simulink model "Model"  (R2023b)
settings: Solver=FixedStepAuto  StartTime=0.0  StopTime=10  FixedStep=0.002  RelTol=1e-3
model workspace (MAT data in the model file):
  a = 0
undefined symbols (not defined in the file or in its folder): X, Y, Z
libraries: sm_lib x84, nesl_utility x29, slpidlib x9, simulink x6
(part 6 of 7)

== matlab function Model/左腿VMC ==
  data: phi_1 input; phi_4 input; F input; T1 output; T2 output; Tp input
function [T1,T2]= fcn(phi_1,phi_4,F,Tp)

l_1=0.15;
l_2=0.27;
l_3=0.27;
l_4=0.15;
l_5=0.15;

J11=(2*(l_1*cos(phi_1) + (2*l_2*cos(2*atan(((4*l_2^2*(l_1*sin(phi_1) - l_4*sin(phi_4))^2 - ((l_1*sin(phi_1) - l_4*sin(phi_4))^2 + (l_5 - l_1*cos(phi_1) + l_4*cos(phi_4))^2 + l_2^2 - l_3^2)^2 + 4*l_2^2*(l_5 - l_1*cos(phi_1) + l_4*cos(phi_4))^2)^(1/2) - 2*l_2*(l_1*sin(phi_1) - l_4*sin(phi_4)))/((l_1*sin(phi_1) - l_4*sin(phi_4))^2 + (l_5 - l_1*cos(phi_1) + l_4*cos(phi_4))^2 + l_2^2 - l_3^2 + 2*l_2*(l_5 - l_1*cos(phi_1) + l_4*cos(phi_4)))))*(((8*l_1*l_2^2*cos(phi_1)*(l_1*sin(phi_1) - l_4*sin(phi_4)) - 2*(2*l_1*cos(phi_1)*(l_1*sin(phi_1) - l_4*sin(phi_4)) + 2*l_1*sin(phi_1)*(l_5 - l_1*cos(phi_1) + l_4*cos(phi_4)))*((l_1*sin(phi_1) - l_4*sin(phi_4))^2 + (l_5 - l_1*cos(phi_1) + l_4*cos(phi_4))^2 + l_2^2 - l_3^2) + 8*l_1*l_2^2*sin(phi_1)*(l_5 - l_1*cos(phi_1) + l_4*cos(phi_4)))/(2*(4*l_2^2*(l_1*sin(phi_1) - l_4*sin(phi_4))^2 - ((l_1*sin(phi_1) - l_4*sin(phi_4))^2 + (l_5 - l_1*cos(phi_1) + l_4*cos(phi_4))^2 + l_2^2 - l_3^2)^2 + 4*l_2^2*(l_5 - l_1*cos(phi_1) + l_4*cos(phi_4))^2)^(1/2)) - 2*l_1*l_2*cos(phi_1))/((l_1*sin(phi_1) - l_4*sin(phi_4))^2 + (l_5 - l_1*cos(phi_1) + l_4*cos(phi_4))^2 + l_2^2 - l_3^2 + 2*l_2*(l_5 - l_1*cos(phi_1) + l_4*cos(phi_4))) - (((4*l_2^2*(l_1*sin(phi_1) - l_4*sin(phi_4))^2 - ((l_1*sin(phi_1) - l_4*sin(phi_4))^2 + (l_5 - l_1*cos(phi_1) + l_4*cos(phi_4))^2 + l_2^2 - l_3^2)^2 + 4*l_2^2*(l_5 - l_1*cos(phi_1) + l_4*cos(phi_4))^2)^(1/2) - 2*l_2*(l_1*sin(phi_1) - l_4*sin(phi_4)))*(2*l_1*l_2*sin(phi_1) + 2*l_1*cos(phi_1)*(l_1*sin(phi_1) - l_4*sin(phi_4)) + 2*l_1*sin(phi_1)*(l_5 - l_1*cos(phi_1) + l_4*cos(phi_4))))/((l_1*sin(phi_1) - l_4*sin(phi_4))^2 + (l_5 - l_1*cos(phi_1) + l_4*cos(phi_4))^2 + l_2^2 - l_3^2 + 2*l_2*(l_5 - l_1*cos(phi_1) + l_4*cos(phi_4)))^2))/(((4*l_2^2*(l_1*sin(phi_1) - l_4*sin(phi_4))^2 - ((l_1*sin(phi_1) - l_4*sin(phi_4))^2 + (l_5 - l_1*cos(phi_1) + l_4*cos(phi_4))^2 + l_2^2 - l_3^2)^2 + 4*l_2^2*(l_5 - l_1*cos(phi_1) + l_4*cos(phi_4))^2)^(1/2) - 2*l_2*(l_1*sin(phi_1) - l_4*sin(phi_4)))^2/((l_1*sin(phi_1) - l_4*sin(phi_4))^2 + (l_5 - l_1*cos(phi_1) + l_4*cos(phi_4))^2 + l_2^2 - l_3^2 + 2*l_2*(l_5 - l_1*cos(phi_1) + l_4*cos(phi_4)))^2 + 1))*(l_2*sin(2*atan(((4*l_2^2*(l_1*sin(phi_1) - l_4*sin(phi_4))^2 - ((l_1*sin(phi_1) - l_4*sin(phi_4))^2 + (l_5 - l_1*cos(phi_1) + l_4*cos(phi_4))^2 + l_2^2 - l_3^2)^2 + 4*l_2^2*(l_5 - l_1*cos(phi_1) + l_4*cos(phi_4))^2)^(1/2) - 2*l_2*(l_1*sin(phi_1) - l_4*sin(phi_4)))/((l_1*sin(phi_1) - l_4*sin(phi_4))^2 + (l_5 - l_1*cos(phi_1) + l_4*cos(phi_4))^2 + l_2^2 - l_3^2 + 2*l_2*(l_5 - l_1*cos(phi_1) + l_4*cos(phi_4))))) + l_1*sin(phi_1)) - 2*(l_1*sin(phi_1) + (2*l_2*sin(2*atan(((4*l_2^2*(l_1*sin(phi_1) - l_4*sin(phi_4))^2 - ((l_1*sin(phi_1) - l_4*sin(phi_4))^2 + (l_5 - l_1*cos(phi_1) + l_4*cos(phi_4))^2 + l_2^2 - l_3^2)^2 + 4*l_2^2*(l_5 - l_1*cos(phi_1) + l_4*cos(phi_4))^2)^(1/2) - 2*l_2*(l_1*sin(phi_1) - l_4*sin(phi_4)))/((l_1*sin(phi_1) - l_4*sin(phi_4))^2 + (l_5 - l_1*cos(phi_1) + l_4*cos(phi_4))^2 + l_2^2 - l_3^2 + 2*l_2*(l_5 - l_1*cos(phi_1) + l_4*cos(phi_4)))))*(((8*l_1*l_2^2*cos(phi_1)*(l_1*sin(phi_1) - l_4*sin(phi_4)) - 2*(2*l_1*cos(phi_1)*(l_1*sin(phi_1) - l_4*sin(phi_4)) + 2*l_1*sin(phi_1)*(l_5 - l_1*cos(phi_1) + l_4*cos(phi_4)))*((l_1*sin(phi_1) - l_4*sin(phi_4))^2 + (l_5 - l_1*cos(phi_1) + l_4*cos(phi_4))^2 + l_2^2 - l_3^2) + 8*l_1*l_2^2*sin(phi_1)*(l_5 - l_1*cos(phi_1) + l_4*cos(phi_4)))/(2*(4*l_2^2*(l_1*sin(phi_1) - l_4*sin(phi_4))^2 - ((l_1*sin(phi_1) - l_4*sin(phi_4))^2 + (l_5 - l_1*cos(phi_1) + l_4*cos(phi_4))^2 + l_2^2 - l_3^2)^2 + 4*l_2^2*(l_5 - l_1*cos(phi_1) + l_4*cos(phi_4))^2)^(1/2)) - 2*l_1*l_2*cos(phi_1))/((l_1*sin(phi_1) - l_4*sin(phi_4))^2 + (l_5 - l_1*cos(phi_1) + l_4*cos(phi_4))^2 + l_2^2 - l_3^2 + 2*l_2*(l_5 - l_1*cos(phi_1) + l_4*cos(phi_4))) - (((4*l_2^2*(l_1*sin(phi_1) - l_4*sin(phi_4))^2 - ((l_1*sin(phi_1) - l_4*sin(phi_4))^2 + (l_5 - l_1*cos(phi_1) + l_4*cos(phi_4))^2 + l_2^2 - l_3^2)^2 + 4*l_2^2*(l_5 - l_1*cos(phi_1) + l_4*cos(phi_4))^2)^(1/2) - 2*l_2*(l_1*sin(phi_1) - l_4*sin(phi_4)))*(2*l_1*l_2*sin(phi_1) + 2*l_1*cos(phi_1)*(l_1*sin(phi_1) - l_4*sin(phi_4)) + 2*l_1*sin(phi_1)*(l_5 - l_1*cos(phi_1) + l_4*cos(phi_4))))/((l_1*sin(phi_1) - l_4*sin(phi_4))^2 + (l_5 - l_1*cos(phi_1) + l_4*cos(phi_4))^2 + l_2^2 - l_3^2 + 2*l_2*(l_5 - l_1*cos(phi_1) + l_4*cos(phi_4)))^2))/(((4*l_2^2*(l_1*sin(phi_1) - l_4*sin(phi_4))^2 - ((l_1*sin(phi_1) - l_4*sin(phi_4))^2 + (l_5 - l_1*cos(phi_1) + l_4*cos(phi_4))^2 + l_2^2 - l_3^2)^2 + 4*l_2^2*(l_5 - l_1*cos(phi_1) + l_4*cos(phi_4))^2)^(1/2) - 2*l_2*(l_1*sin(phi_1) - l_4*sin(phi_4)))^2/((l_1*sin(phi_1) - l_4*sin(phi_4))^2 + (l_5 - l_1*cos(phi_1) + l_4*cos(phi_4))^2 + l_2^2 - l_3^2 + 2*l_2*(l_5 - l_1*cos(phi_1) + l_4*cos(phi_4)))^2 + 1))*(l_2*cos(2*atan(((4*l_2^2*(l_1*sin(phi_1) - l_4*sin(phi_4))^2 - ((l_1*sin(phi_1) - l_4*sin(phi_4))^2 + (l_5 - l_1*cos(phi_1) + l_4*cos(phi_4))^2 + l_2^2 - l_3^2)^2 + 4*l_2^2*(l_5 - l_1*cos(phi_1) + l_4*cos(phi_4))^2)^(1/2) - 2*l_2*(l_1*sin(phi_1) - l_4*sin(phi_4)))/((l_1*sin(phi_1) - l_4*sin(phi_4))^2 + (l_5 - l_1*cos(phi_1) + l_4*cos(phi_4))^2 + l_2^2 - l_3^2 + 2*l_2*(l_5 - l_1*cos(phi_1) + l_4*cos(phi_4))))) - l_5/2 + l_1*cos(phi_1)))/(2*((l_2*sin(2*atan(((4*l_2^2*(l_1*sin(phi_1) - l_4*sin(phi_4))^2 - ((l_1*sin(phi_1) - l_4*sin(phi_4))^2 + (l_5 - l_1*cos(phi_1) + l_4*cos(phi_4))^2 + l_2^2 - l_3^2)^2 + 4*l_2^2*(l_5 - l_1*cos(phi_1) + l_4*cos(phi_4))^2)^(1/2) - 2*l_2*(l_1*sin(phi_1) - l_4*sin(phi_4)))/((l_1*sin(phi_1) - l_4*sin(phi_4))^2 + (l_5 - l_1*cos(phi_1) + l_4*cos(phi_4))^2 + l_2^2 - l_3^2 + 2*l_2*(l_5 - l_1*cos(phi_1) + l_4*cos(phi_4))))) + l_1*sin(phi_1))^2 + (l_2*cos(2*atan(((4*l_2^2*(l_1*sin(phi_1) - l_4*sin(phi_4))^2 - ((l_1*sin(phi_1) - l_4*sin(phi_4))^2 + (l_5 - l_1*cos(phi_1) + l_4*cos(phi_4))^2 + l_2^2 - l_3^2)^2 + 4*l_2^2*(l_5 - l_1*cos(phi_1) + l_4*cos(phi_4))^2)^(1/2) - 2*l_2*(l_1*sin(phi_1) - l_4*sin(phi_4)))/((l_1*sin(phi_1) - l_4*sin(phi_4))^2 + (l_5 - l_1*cos(phi_1) + l_4*cos(phi_4))^2 + l_2^2 - l_3^2 + 2*l_2*(l_5 - l_1*cos(phi_1) + l_4*cos(phi_4))))) - l_5/2 + l_1*cos(phi_1))^2)^(1/2));
J12=((4*l_2*sin(2*atan(((4*l_2^2*(l_1*sin(phi_1) - l_4*sin(phi_4))^2 - ((l_1*sin(phi_1) - l_4*sin(phi_4))^2 + (l_5 - l_1*cos(phi_1) + l_4*cos(phi_4))^2 + l_2^2 - l_3^2)^2 + 4*l_2^2*(l_5 - l_1*cos(phi_1) + l_4*cos(phi_4))^2)^(1/2) - 2*l_2*(l_1*sin(phi_1) - l_4*sin(phi_4)))/((l_1*sin(phi_1) - l_4*sin(phi_4))^2 + (l_5 - l_1*cos(phi_1) + l_4*cos(phi_4))^2 + l_2^2 - l_3^2 + 2*l_2*(l_5 - l_1*cos(phi_1) + l_4*cos(phi_4)))))*(((8*l_2^2*l_4*cos(phi_4)*(l_1*sin(phi_1) - l_4*sin(phi_4)) - 2*(2*l_4*cos(phi_4)*(l_1*sin(phi_1) - l_4*sin(phi_4)) + 2*l_4*sin(phi_4)*(l_5 - l_1*cos(phi_1) + l_4*cos(phi_4)))*((l_1*sin(phi_1) - l_4*sin(phi_4))^2 + (l_5 - l_1*cos(phi_1) + l_4*cos(phi_4))^2 + l_2^2 - l_3^2) + 8*l_2^2*l_4*sin(phi_4)*(l_5 - l_1*cos(phi_1) + l_4*cos(phi_4)))/(2*(4*l_2^2*(l_1*sin(phi_1) - l_4*sin(phi_4))^2 - ((l_1*sin(phi_1) - l_4*sin(phi_4))^2 + (l_5 - l_1*cos(phi_1) + l_4*cos(phi_4))^2 + l_2^2 - l_3^2)^2 + 4*l_2^2*(l_5 - l_1*cos(phi_1) + l_4*cos(phi_4))^2)^(1/2)) - 2*l_2*l_4*cos(phi_4))/((l_1*sin(phi_1) - l_4*sin(phi_4))^2 + (l_5 - l_1*cos(phi_1) + l_4*cos(phi_4))^2 + l_2^2 - l_3^2 + 2*l_2*(l_5 - l_1*cos(phi_1) + l_4*cos(phi_4))) - (((4*l_2^2*(l_1*sin(phi_1) - l_4*sin(phi_4))^2 - ((l_1*sin(phi_1) - l_4*sin(phi_4))^2 + (l_5 - l_1*cos(phi_1) + l_4*cos(phi_4))^2 + l_2^2 - l_3^2)^2 + 4*l_2^2*(l_5 - l_1*cos(phi_1) + l_4*cos(phi_4))^2)^(1/2) - 2*l_2*(l_1*sin(phi_1) - l_4*sin(phi_4)))*(2*l_2*l_4*sin(phi_4) + 2*l_4*cos(phi_4)*(l_1*sin(phi_1) - l_4*sin(phi_4)) + 2*l_4*sin(phi_4)*(l_5 - l_1*cos(phi_1) + l_4*cos(phi_4))))/((l_1*sin(phi_1) - l_4*sin(phi_4))^2 + (l_5 - l_1*cos(phi_1) + l_4*cos(phi_4))^2 + l_2^2 - l_3^2 + 2*l_2*(l_5 - l_1*cos(phi_1) + l_4*cos(phi_4)))^2)*(l_2*cos(2*atan(((4*l_2^2*(l_1*sin(phi_1) - l_4*sin(phi_4))^2 - ((l_1*sin(phi_1) - l_4*sin(phi_4))^2 + (l_5 - l_1*cos(phi_1) + l_4*cos(phi_4))^2 + l_2^2 - l_3^2)^2 + 4*l_2^2*(l_5 - l_1*cos(phi_1) + l_4*cos(phi_4))^2)^(1/2) - 2*l_2*(l_1*sin(phi_1) - l_4*sin(phi_4)))/((l_1*sin(phi_1) - l_4*sin(phi_4))^2 + (l_5 - l_1*cos(phi_1) + l_4*cos(phi_4))^2 + l_2^2 - l_3^2 + 2*l_2*(l_5 - l_1*cos(phi_1) + l_4*cos(phi_4))))) - l_5/2 + l_1*cos(phi_1)))/(((4*l_2^2*(l_1*sin(phi_1) - l_4*sin(phi_4))^2 - ((l_1*sin(phi_1) - l_4*sin(phi_4))^2 + (l_5 - l_1*cos(phi_1) + l_4*cos(phi_4))^2 + l_2^2 - l_3^2)^2 + 4*l_2^2*(l_5 - l_1*cos(phi_1) + l_4*cos(phi_4))^2)^(1/2) - 2*l_2*(l_1*sin(phi_1) - l_4*sin(phi_4)))^2/((l_1*sin(phi_1) - l_4*sin(phi_4))^2 + (l_5 - l_1*cos(phi_1) + l_4*cos(phi_4))^2 + l_2^2 - l_3^2 + 2*l_2*(l_5 - l_1*cos(phi_1) + l_4*cos(phi_4)))^2 + 1) - (4*l_2*cos(2*atan(((4*l_2^2*(l_1*sin(phi_1) - l_4*sin(phi_4))^2 - ((l_1*sin(phi_1) - l_4*sin(phi_4))^2 + (l_5 - l_1*cos(phi_1) + l_4*cos(phi_4))^2 + l_2^2 - l_3^2)^2 + 4*l_2^2*(l_5 - l_1*cos(phi_1) + l_4*cos(phi_4))^2)^(1/2) - 2*l_2*(l_1*sin(phi_1) - l_4*sin(phi_4)))/((l_1*sin(phi_1) - l_4*sin(phi_4))^2 + (l_5 - l_1*cos(phi_1) + l_4*cos(phi_4))^2 + l_2^2 - l_3^2 + 2*l_2*(l_5 - l_1*cos(phi_1) + l_4*cos(phi_4)))))*(l_2*sin(2*atan(((4*l_2^2*(l_1*sin(phi_1) - l_4*sin(phi_4))^2 - ((l_1*sin(phi_1) - l_4*sin(phi_4))^2 + (l_5 - l_1*cos(phi_1) + l_4*cos(phi_4))^2 + l_2^2 - l_3^2)^2 + 4*l_2^2*(l_5 - l_1*cos(phi_1) + l_4*cos(phi_4))^2)^(1/2) - 2*l_2*(l_1*sin(phi_1) - l_4*sin(phi_4)))/((l_1*sin(phi_1) - l_4*sin(phi_4))^2 + (l_5 - l_1*cos(phi_1) + l_4*cos(phi_4))^2 + l_2^2 - l_3^2 + 2*l_2*(l_5 - l_1*cos(phi_1) + l_4*cos(phi_4))))) + l_1*sin(phi_1))*(((8*l_2^2*l_4*cos(phi_4)*(l_1*sin(phi_1) - l_4*sin(phi_4)) - 2*(2*l_4*cos(phi_4)*(l_1*sin(phi_1) - l_4*sin(phi_4)) + 2*l_4*sin(phi_4)*(l_5 - l_1*cos(phi_1) + l_4*cos(phi_4)))*((l_1*sin(phi_1) - l_4*sin(phi_4))^2 + (l_5 - l_1*cos(phi_1) + l_4*cos(phi_4))^2 + l_2^2 - l_3^2) + 8*l_2^2*l_4*sin(phi_4)*(l_5 - l_1*cos(phi_1) + l_4*cos(phi_4)))/(2*(4*l_2^2*(l_1*sin(phi_1) - l_4*sin(phi_4))^2 - ((l_1*sin(phi_1) - l_4*sin(phi_4))^2 + (l_5 - l_1*cos(phi_1) + l_4*cos(phi_4))^2 + l_2^2 - l_3^2)^2 + 4*l_2^2*(l_5 - l_1*cos(phi_1) + l_4*cos(phi_4))^2)^(1/2)) - 2*l_2*l_4*cos(phi_4))/((l_1*sin(phi_1) - l_4*sin(phi_4))^2 + (l_5 - l_1*cos(phi_1) + l_4*cos(phi_4))^2 + l_2^2 - l_3^2 + 2*l_2*(l_5 - l_1*cos(phi_1) + l_4*cos(phi_4))) - (((4*l_2^2*(l_1*sin(phi_1) - l_4*sin(phi_4))^2 - ((l_1*sin(phi_1) - l_4*sin(phi_4))^2 + (l_5 - l_1*cos(phi_1) + l_4*cos(phi_4))^2 + l_2^2 - l_3^2)^2 + 4*l_2^2*(l_5 - l_1*cos(phi_1) + l_4*cos(phi_4))^2)^(1/2) - 2*l_2*(l_1*sin(phi_1) - l_4*sin(phi_4)))*(2*l_2*l_4*sin(phi_4) + 2*l_4*cos(phi_4)*(l_1*sin(phi_1) - l_4*sin(phi_4)) + 2*l_4*sin(phi_4)*(l_5 - l_1*cos(phi_1) + l_4*cos(phi_4))))/((l_1*sin(phi_1) - l_4*sin(phi_4))^2 + (l_5 - l_1*cos(phi_1) + l_4*cos(phi_4))^2 + l_2^2 - l_3^2 + 2*l_2*(l_5 - l_1*cos(phi_1) + l_4*cos(phi_4)))^2))/(((4*l_2^2*(l_1*sin(phi_1) - l_4*sin(phi_4))^2 - ((l_1*sin(phi_1) - l_4*sin(phi_4))^2 + (l_5 - l_1*cos(phi_1) + l_4*cos(phi_4))^2 + l_2^2 - l_3^2)^2 + 4*l_2^2*(l_5 - l_1*cos(phi_1) + l_4*cos(phi_4))^2)^(1/2) - 2*l_2*(l_1*sin(phi_1) - l_4*sin(phi_4)))^2/((l_1*sin(phi_1) - l_4*sin(phi_4))^2 + (l_5 - l_1*cos(phi_1) + l_4*cos(phi_4))^2 + l_2^2 - l_3^2 + 2*l_2*(l_5 - l_1*cos(phi_1) + l_4*cos(phi_4)))^2 + 1))/(2*((l_2*sin(2*atan(((4*l_2^2*(l_1*sin(phi_1) - l_4*sin(phi_4))^2 - ((l_1*sin(phi_1) - l_4*sin(phi_4))^2 + (l_5 - l_1*cos(phi_1) + l_4*cos(phi_4))^2 + l_2^2 - l_3^2)^2 + 4*l_2^2*(l_5 - l_1*cos(phi_1) + l_4*cos(phi_4))^2)^(1/2) - 2*l_2*(l_1*sin(phi_1) - l_4*sin(phi_4)))/((l_1*sin(phi_1) - l_4*sin(phi_4))^2 + (l_5 - l_1*cos(phi_1) + l_4*cos(phi_4))^2 + l_2^2 - l_3^2 + 2*l_2*(l_5 - l_1*cos(phi_1) + l_4*cos(phi_4))))) + l_1*sin(phi_1))^2 + (l_2*cos(2*atan(((4*l_2^2*(l_1*sin(phi_1) - l_4*sin(phi_4))^2 - ((l_1*sin(phi_1) - l_4*sin(phi_4))^2 + (l_5 - l_1*cos(phi_1) + l_4*cos(phi_4))^2 + l_2^2 - l_3^2)^2 + 4*l_2^2*(l_5 - l_1*cos(phi_1) + l_4*cos(phi_4))^2)^(1/2) - 2*l_2*(l_1*sin(phi_1) - l_4*sin(phi_4)))/((l_1*sin(phi_1) - l_4*sin(phi_4))^2 + (l_5 - l_1*cos(phi_1) + l_4*cos(phi_4))^2 + l_2^2 - l_3^2 + 2*l_2*(l_5 - l_1*cos(phi_1) + l_4*cos(phi_4))))) - l_5/2 + l_1*cos(phi_1))^2)^(1/2));
J21=((l_1*sin(phi_1) + (2*l_2*sin(2*atan(((4*l_2^2*(l_1*sin(phi_1) - l_4*sin(phi_4))^2 - ((l_1*sin(phi_1) - l_4*sin(phi_4))^2 + (l_5 - l_1*cos(phi_1) + l_4*cos(phi_4))^2 + l_2^2 - l_3^2)^2 + 4*l_2^2*(l_5 - l_1*cos(phi_1) + l_4*cos(phi_4))^2)^(1/2) - 2*l_2*(l_1*sin(phi_1) - l_4*sin(phi_4)))/((l_1*sin(phi_1) - l_4*sin(phi_4))^2 + (l_5 - l_1*cos(phi_1) + l_4*cos(phi_4))^2 + l_2^2 - l_3^2 + 2*l_2*(l_5 - l_1*cos(phi_1) + l_4*cos(phi_4)))))*(((8*l_1*l_2^2*cos(phi_1)*(l_1*sin(phi_1) - l_4*sin(phi_4)) - 2*(2*l_1*cos(phi_1)*(l_1*sin(phi_1) - l_4*sin(phi_4)) + 2*l_1*sin(phi_1)*(l_5 - l_1*cos(phi_1) + l_4*cos(phi_4)))*((l_1*sin(phi_1) - l_4*sin(phi_4))^2 + (l_5 - l_1*cos(phi_1) + l_4*cos(phi_4))^2 + l_2^2 - l_3^2) + 8*l_1*l_2^2*sin(phi_1)*(l_5 - l_1*cos(phi_1) + l_4*cos(phi_4)))/(2*(4*l_2^2*(l_1*sin(phi_1) - l_4*sin(phi_4))^2 - ((l_1*sin(phi_1) - l_4*sin(phi_4))^2 + (l_5 - l_1*cos(phi_1) + l_4*cos(phi_4))^2 + l_2^2 - l_3^2)^2 + 4*l_2^2*(l_5 - l_1*cos(phi_1) + l_4*cos(phi_4))^2)^(1/2)) - 2*l_1*l_2*cos(phi_1))/((l_1*sin(phi_1) - l_4*sin(phi_4))^2 + (l_5 - l_1*cos(phi_1) + l_4*cos(phi_4))^2 + l_2^2 - l_3^2 + 2*l_2*(l_5 - l_1*cos(phi_1) + l_4*cos(phi_4))) - (((4*l_2^2*(l_1*sin(phi_1) - l_4*sin(phi_4))^2 - ((l_1*sin(phi_1) - l_4*sin(phi_4))^2 + (l_5 - l_1*cos(phi_1) + l_4*cos(phi_4))^2 + l_2^2 - l_3^2)^2 + 4*l_2^2*(l_5 - l_1*cos(phi_1) + l_4*cos(phi_4))^2)^(1/2) - 2*l_2*(l_1*sin(phi_1) - l_4*sin(phi_4)))*(2*l_1*l_2*sin(phi_1) + 2*l_1*cos(phi_1)*(l_1*sin(phi_1) - l_4*sin(phi_4)) + 2*l_1*sin(phi_1)*(l_5 - l_1*cos(phi_1) + l_4*cos(phi_4))))/((l_1*sin(phi_1) - l_4*sin(phi_4))^2 + (l_5 - l_1*cos(phi_1) + l_4*cos(phi_4))^2 + l_2^2 - l_3^2 + 2*l_2*(l_5 - l_1*cos(phi_1) + l_4*cos(phi_4)))^2))/(((4*l_2^2*(l_1*sin(phi_1) - l_4*sin(phi_4))^2 - ((l_1*sin(phi_1) - l_4*sin(phi_4))^2 + (l_5 - l_1*cos(phi_1) + l_4*cos(phi_4))^2 + l_2^2 - l_3^2)^2 + 4*l_2^2*(l_5 - l_1*cos(phi_1) + l_4*cos(phi_4))^2)^(1/2) - 2*l_2*(l_1*sin(phi_1) - l_4*sin(phi_4)))^2/((l_1*sin(phi_1) - l_4*sin(phi_4))^2 + (l_5 - l_1*cos(phi_1) + l_4*cos(phi_4))^2 + l_2^2 - l_3^2 + 2*l_2*(l_5 - l_1*cos(phi_1) + l_4*cos(phi_4)))^2 + 1))/((l_2*sin(2*atan(((4*l_2^2*(l_1*sin(phi_1) - l_4*sin(phi_4))^2 - ((l_1*sin(phi_1) - l_4*sin(phi_4))^2 + (l_5 - l_1*cos(phi_1) + l_4*cos(phi_4))^2 + l_2^2 - l_3^2)^2 + 4*l_2^2*(l_5 - l_1*cos(phi_1) + l_4*cos(phi_4))^2)^(1/2) - 2*l_2*(l_1*sin(phi_1) - l_4*sin(phi_4)))/((l_1*sin(phi_1) - l_4*sin(phi_4))^2 + (l_5 - l_1*cos(phi_1) + l_4*cos(phi_4))^2 + l_2^2 - l_3^2 + 2*l_2*(l_5 - l_1*cos(phi_1) + l_4*cos(phi_4))))) + l_1*sin(phi_1))^2 + (l_2*cos(2*atan(((4*l_2^2*(l_1*sin(phi_1) - l_4*sin(phi_4))^2 - ((l_1*sin(phi_1) - l_4*sin(phi_4))^2 + (l_5 - l_1*cos(phi_1) + l_4*cos(phi_4))^2 + l_2^2 - l_3^2)^2 + 4*l_2^2*(l_5 - l_1*cos(phi_1) + l_4*cos(phi_4))^2)^(1/2) - 2*l_2*(l_1*sin(phi_1) - l_4*sin(phi_4)))/((l_1*sin(phi_1) - l_4*sin(phi_4))^2 + (l_5 - l_1*cos(phi_1) + l_4*cos(phi_4))^2 + l_2^2 - l_3^2 + 2*l_2*(l_5 - l_1*cos(phi_1) + l_4*cos(phi_4))))) - l_5/2 + l_1*cos(phi_1))^2)^(1/2) + ((2*(l_1*cos(phi_1) + (2*l_2*cos(2*atan(((4*l_2^2*(l_1*sin(phi_1) - l_4*sin(phi_4))^2 - ((l_1*sin(phi_1) - l_4*sin(phi_4))^2 + (l_5 - l_1*cos(phi_1) + l_4*cos(phi_4))^2 + l_2^2 - l_3^2)^2 + 4*l_2^2*(l_5 - l_1*cos(phi_1) + l_4*cos(phi_4))^2)^(1/2) - 2*l_2*(l_1*sin(phi_1) - l_4*sin(phi_4)))/((l_1*sin(phi_1) - l_4*sin(phi_4))^2 + (l_5 - l_1*cos(phi_1) + l_4*cos(phi_4))^2 + l_2^2 - l_3^2 + 2*l_2*(l_5 - l_1*cos(phi_1) + l_4*cos(phi_4)))))*(((8*l_1*l_2^2*cos(phi_1)*(l_1*sin(phi_1) - l_4*sin(phi_4)) - 2*(2*l_1*cos(phi_1)*(l_1*sin(phi_1) - l_4*sin(phi_4)) + 2*l_1*sin(phi_1)*(l_5 - l_1*cos(phi_1) + l_4*cos(phi_4)))*((l_1*sin(phi_1) - l_4*sin(phi_4))^2 + (l_5 - l_1*cos(phi_1) + l_4*cos(phi_4))^2 + l_2^2 - l_3^2) + 8*l_1*l_2^2*sin(phi_1)*(l_5 - l_1*cos(phi_1) + l_4*cos(phi_4)))/(2*(4*l_2^2*(l_1*sin(phi_1) - l_4*sin(phi_4))^2 - ((l_1*sin(phi_1) - l_4*sin(phi_4))^2 + (l_5 - l_1*cos(phi_1) + l_4*cos(phi_4))^2 + l_2^2 - l_3^2)^2 + 4*l_2^2*(l_5 - l_1*cos(phi_1) + l_4*cos(phi_4))^2)^(1/2)) - 2*l_1*l_2*cos(phi_1))/((l_1*sin(phi_1) - l_4*sin(phi_4))^2 + (l_5 - l_1*cos(phi_1) + l_4*cos(phi_4))^2 + l_2^2 - l_3^2 + 2*l_2*(l_5 - l_1*cos(phi_1) + l_4*cos(phi_4))) - (((4*l_2^2*(l_1*sin(phi_1) - l_4*sin(phi_4))^2 - ((l_1*sin(phi_1) - l_4*sin(phi_4))^2 + (l_5 - l_1*cos(phi_1) + l_4*cos(phi_4))^2 + l_2^2 - l_3^2)^2 + 4*l_2^2*(l_5 - l_1*cos(phi_1) + l_4*cos(phi_4))^2)^(1/2) - 2*l_2*(l_1*sin(phi_1) - l_4*sin(phi_4)))*(2*l_1*l_2*sin(phi_1) + 2*l_1*cos(phi_1)*(l_1*sin(phi_1) - l_4*sin(phi_4)) + 2*l_1*sin(phi_1)*(l_5 - l_1*cos(phi_1) + l_4*cos(phi_4))))/((l_1*sin(phi_1) - l_4*sin(phi_4))^2 + (l_5 - l_1*cos(phi_1) + l_4*cos(phi_4))^2 + l_2^2 - l_3^2 + 2*l_2*(l_5 - l_1*cos(phi_1) + l_4*cos(phi_4)))^2))/(((4*l_2^2*(l_1*sin(phi_1) - l_4*sin(phi_4))^2 - ((l_1*sin(phi_1) - l_4*sin(phi_4))^2 + (l_5 - l_1*cos(phi_1) + l_4*cos(phi_4))^2 + l_2^2 - l_3^2)^2 + 4*l_2^2*(l_5 - l_1*cos(phi_1) + l_4*cos(phi_4))^2)^(1/2) - 2*l_2*(l_1*sin(phi_1) - l_4*sin(phi_4)))^2/((l_1*sin(phi_1) - l_4*sin(phi_4))^2 + (l_5 - l_1*cos(phi_1) + l_4*cos(phi_4))^2 + l_2^2 - l_3^2 + 2*l_2*(l_5 - l_1*cos(phi_1) + l_4*cos(phi_4)))^2 + 1))*(l_2*sin(2*atan(((4*l_2^2*(l_1*sin(phi_1) - l_4*sin(phi_4))^2 - ((l_1*sin(phi_1) - l_4*sin(phi_4))^2 + (l_5 - l_1*cos(phi_1) + l_4*cos(phi_4))^2 + l_2^2 - l_3^2)^2 + 4*l_2^2*(l_5 - l_1*cos(phi_1) + l_4*cos(phi_4))^2)^(1/2) - 2*l_2*(l_1*sin(phi_1) - l_4*sin(phi_4)))/((l_1*sin(phi_1) - l_4*sin(phi_4))^2 + (l_5 - l_1*cos(phi_1) + l_4*cos(phi_4))^2 + l_2^2 - l_3^2 + 2*l_2*(l_5 - l_1*cos(phi_1) + l_4*cos(phi_4))))) + l_1*sin(phi_1)) - 2*(l_1*sin(phi_1) + (2*l_2*sin(2*atan(((4*l_2^2*(l_1*sin(phi_1) - l_4*sin(phi_4))^2 - ((l_1*sin(phi_1) - l_4*sin(phi_4))^2 + (l_5 - l_1*cos(phi_1) + l_4*cos(phi_4))^2 + l_2^2 - l_3^2)^2 + 4*l_2^2*(l_5 - l_1*cos(phi_1) + l_4*cos(phi_4))^2)^(1/2) - 2*l_2*(l_1*sin(phi_1) - l_4*sin(phi_4)))/((l_1*sin(phi_1) - l_4*sin(phi_4))^2 + (l_5 - l_1*cos(phi_1) + l_4*cos(phi_4))^2 + l_2^2 - l_3^2 + 2*l_2*(l_5 - l_1*cos(phi_1) + l_4*cos(phi_4)))))*(((8*l_1*l_2^2*cos(phi_1)*(l_1*sin(phi_1) - l_4*sin(phi_4)) - 2*(2*l_1*cos(phi_1)*(l_1*sin(phi_1) - l_4*sin(phi_4)) + 2*l_1*sin(phi_1)*(l_5 - l_1*cos(phi_1) + l_4*cos(phi_4)))*((l_1*sin(phi_1) - l_4*sin(phi_4))^2 + (l_5 - l_1*cos(phi_1) + l_4*cos(phi_4))^2 + l_2^2 - l_3^2) + 8*l_1*l_2^2*sin(phi_1)*(l_5 - l_1*cos(phi_1) + l_4*cos(phi_4)))/(2*(4*l_2^2*(l_1*sin(phi_1) - l_4*sin(phi_4))^2 - ((l_1*sin(phi_1) - l_4*sin(phi_4))^2 + (l_5 - l_1*cos(phi_1) + l_4*cos(phi_4))^2 + l_2^2 - l_3^2)^2 + 4*l_2^2*(l_5 - l_1*cos(phi_1) + l_4*cos(phi_4))^2)^(1/2)) - 2*l_1*l_2*cos(phi_1))/((l_1*sin(phi_1) - l_4*sin(phi_4))^2 + (l_5 - l_1*cos(phi_1) + l_4*cos(phi_4))^2 + l_2^2 - l_3^2 + 2*l_2*(l_5 - l_1*cos(phi_1) + l_4*cos(phi_4))) - (((4*l_2^2*(l_1*sin(phi_1) - l_4*sin(phi_4))^2 - ((l_1*sin(phi_1) - l_4*sin(phi_4))^2 + (l_5 - l_1*cos(phi_1) + l_4*cos(phi_4))^2 + l_2^2 - l_3^2)^2 + 4*l_2^2*(l_5 - l_1*cos(phi_1) + l_4*cos(phi_4))^2)^(1/2) - 2*l_2*(l_1*sin(phi_1) - l_4*sin(phi_4)))*(2*l_1*l_2*sin(phi_1) + 2*l_1*cos(phi_1)*(l_1*sin(phi_1) - l_4*sin(phi_4)) + 2*l_1*sin(phi_1)*(l_5 - l_1*cos(phi_1) + l_4*cos(phi_4))))/((l_1*sin(phi_1) - l_4*sin(phi_4))^2 + (l_5 - l_1*cos(phi_1) + l_4*cos(phi_4))^2 + l_2^2 - l_3^2 + 2*l_2*(l_5 - l_1*cos(phi_1) + l_4*cos(phi_4)))^2))/(((4*l_2^2*(l_1*sin(phi_1) - l_4*sin(phi_4))^2 - ((l_1*sin(phi_1) - l_4*sin(phi_4))^2 + (l_5 - l_1*cos(phi_1) + l_4*cos(phi_4))^2 + l_2^2 - l_3^2)^2 + 4*l_2^2*(l_5 - l_1*cos(phi_1) + l_4*cos(phi_4))^2)^(1/2) - 2*l_2*(l_1*sin(phi_1) - l_4*sin(phi_4)))^2/((l_1*sin(phi_1) - l_4*sin(phi_4))^2 + (l_5 - l_1*cos(phi_1) + l_4*cos(phi_4))^2 + l_2^2 - l_3^2 + 2*l_2*(l_5 - l_1*cos(phi_1) + l_4*cos(phi_4)))^2 + 1))*(l_2*cos(2*atan(((4*l_2^2*(l_1*sin(phi_1) - l_4*sin(phi_4))^2 - ((l_1*sin(phi_1) - l_4*sin(phi_4))^2 + (l_5 - l_1*cos(phi_1) + l_4*cos(phi_4))^2 + l_2^2 - l_3^2)^2 + 4*l_2^2*(l_5 - l_1*cos(phi_1) + l_4*cos(phi_4))^2)^(1/2) - 2*l_2*(l_1*sin(phi_1) - l_4*sin(phi_4)))/((l_1*sin(phi_1) - l_4*sin(phi_4))^2 + (l_5 - l_1*cos(phi_1) + l_4*cos(phi_4))^2 + l_2^2 - l_3^2 + 2*l_2*(l_5 - l_1*cos(phi_1) + l_4*cos(phi_4))))) - l_5/2 + l_1*cos(phi_1)))*(l_2*cos(2*atan(((4*l_2^2*(l_1*sin(phi_1) - l_4*sin(phi_4))^2 - ((l_1*sin(phi_1) - l_4*sin(phi_4))^2 + (l_5 - l_1*cos(phi_1) + l_4*cos(phi_4))^2 + l_2^2 - l_3^2)^2 + 4*l_2^2*(l_5 - l_1*cos(phi_1) + l_4*cos(phi_4))^2)^(1/2) - 2*l_2*(l_1*sin(phi_1) - l_4*sin(phi_4)))/((l_1*sin(phi_1) - l_4*sin(phi_4))^2 + (l_5 - l_1*cos(phi_1) + l_4*cos(phi_4))^2 + l_2^2 - l_3^2 + 2*l_2*(l_5 - l_1*cos(phi_1) + l_4*cos(phi_4))))) - l_5/2 + l_1*cos(phi_1)))/(2*((l_2*sin(2*atan(((4*l_2^2*(l_1*sin(phi_1) - l_4*sin(phi_4))^2 - ((l_1*sin(phi_1) - l_4*sin(phi_4))^2 + (l_5 - l_1*cos(phi_1) + l_4*cos(phi_4))^2 + l_2^2 - l_3^2)^2 + 4*l_2^2*(l_5 - l_1*cos(phi_1) + l_4*cos(phi_4))^2)^(1/2) - 2*l_2*(l_1*sin(phi_1) - l_4*sin(phi_4)))/((l_1*sin(phi_1) - l_4*sin(phi_4))^2 + (l_5 - l_1*cos(phi_1) + l_4*cos(phi_4))^2 + l_2^2 - l_3^2 + 2*l_2*(l_5 - l_1*cos(phi_1) + l_4*cos(phi_4))))) + l_1*sin(phi_1))^2 + (l_2*cos(2*atan(((4*l_2^2*(l_1*sin(phi_1) - l_4*sin(phi_4))^2 - ((l_1*sin(phi_1) - l_4*sin(phi_4))^2 + (l_5 - l_1*cos(phi_1) + l_4*cos(phi_4))^2 + l_2^2 - l_3^2)^2 + 4*l_2^2*(l_5 - l_1*cos(phi_1) + l_4*cos(phi_4))^2)^(1/2) - 2*l_2*(l_1*sin(phi_1) - l_4*sin(phi_4)))/((l_1*sin(phi_1) - l_4*sin(phi_4))^2 + (l_5 - l_1*cos(phi_1) + l_4*cos(phi_4))^2 + l_2^2 - l_3^2 + 2*l_2*(l_5 - l_1*cos(phi_1) + l_4*cos(phi_4))))) - l_5/2 + l_1*cos(phi_1))^2)^(3/2)))/(1 - (l_2*cos(2*atan(((4*l_2^2*(l_1*sin(phi_1) - l_4*sin(phi_4))^2 - ((l_1*sin(phi_1) - l_4*sin(phi_4))^2 + (l_5 - l_1*cos(phi_1) + l_4*cos(phi_4))^2 + l_2^2 - l_3^2)^2 + 4*l_2^2*(l_5 - l_1*cos(phi_1) + l_4*cos(phi_4))^2)^(1/2) - 2*l_2*(l_1*sin(phi_1) - l_4*sin(phi_4)))/((l_1*sin(phi_1) - l_4*sin(phi_4))^2 + (l_5 - l_1*cos(phi_1) + l_4*cos(phi_4))^2 + l_2^2 - l_3^2 + 2*l_2*(l_5 - l_1*cos(phi_1) + l_4*cos(phi_4))))) - l_5/2 + l_1*cos(phi_1))^2/((l_2*sin(2*atan(((4*l_2^2*(l_1*sin(phi_1) - l_4*sin(phi_4))^2 - ((l_1*sin(phi_1) - l_4*sin(phi_4))^2 + (l_5 - l_1*cos(phi_1) + l_4*cos(phi_4))^2 + l_2^2 - l_3^2)^2 + 4*l_2^2*(l_5 - l_1*cos(phi_1) + l_4*cos(phi_4))^2)^(1/2) - 2*l_2*(l_1*sin(phi_1) - l_4*sin(phi_4)))/((l_1*sin(phi_1) - l_4*sin(phi_4))^2 + (l_5 - l_1*cos(phi_1) + l_4*cos(phi_4))^2 + l_2^2 - l_3^2 + 2*l_2*(l_5 - l_1*cos(phi_1) + l_4*cos(phi_4))))) + l_1*sin(phi_1))^2 + (l_2*cos(2*atan(((4*l_2^2*(l_1*sin(phi_1) - l_4*sin(phi_4))^2 - ((l_1*sin(phi_1) - l_4*sin(phi_4))^2 + (l_5 - l_1*cos(phi_1) + l_4*cos(phi_4))^2 + l_2^2 - l_3^2)^2 + 4*l_2^2*(l_5 - l_1*cos(phi_1) + l_4*cos(phi_4))^2)^(1/2) - 2*l_2*(l_1*sin(phi_1) - l_4*sin(phi_4)))/((l_1*sin(phi_1) - l_4*sin(phi_4))^2 + (l_5 - l_1*cos(phi_1) + l_4*cos(phi_4))^2 + l_2^2 - l_3^2 + 2*l_2*(l_5 - l_1*cos(phi_1) + l_4*cos(phi_4))))) - l_5/2 + l_1*cos(phi_1))^2))^(1/2);
J22=((((4*l_2*sin(2*atan(((4*l_2^2*(l_1*sin(phi_1) - l_4*sin(phi_4))^2 - ((l_1*sin(phi_1) - l_4*sin(phi_4))^2 + (l_5 - l_1*cos(phi_1) + l_4*cos(phi_4))^2 + l_2^2 - l_3^2)^2 + 4*l_2^2*(l_5 - l_1*cos(phi_1) + l_4*cos(phi_4))^2)^(1/2) - 2*l_2*(l_1*sin(phi_1) - l_4*sin(phi_4)))/((l_1*sin(phi_1) - l_4*sin(phi_4))^2 + (l_5 - l_1*cos(phi_1) + l_4*cos(phi_4))^2 + l_2^2 - l_3^2 + 2*l_2*(l_5 - l_1*cos(phi_1) + l_4*cos(phi_4)))))*(((8*l_2^2*l_4*cos(phi_4)*(l_1*sin(phi_1) - l_4*sin(phi_4)) - 2*(2*l_4*cos(phi_4)*(l_1*sin(phi_1) - l_4*sin(phi_4)) + 2*l_4*sin(phi_4)*(l_5 - l_1*cos(phi_1) + l_4*cos(phi_4)))*((l_1*sin(phi_1) - l_4*sin(phi_4))^2 + (l_5 - l_1*cos(phi_1) + l_4*cos(phi_4))^2 + l_2^2 - l_3^2) + 8*l_2^2*l_4*sin(phi_4)*(l_5 - l_1*cos(phi_1) + l_4*cos(phi_4)))/(2*(4*l_2^2*(l_1*sin(phi_1) - l_4*sin(phi_4))^2 - ((l_1*sin(phi_1) - l_4*sin(phi_4))^2 + (l_5 - l_1*cos(phi_1) + l_4*cos(phi_4))^2 + l_2^2 - l_3^2)^2 + 4*l_2^2*(l_5 - l_1*cos(phi_1) + l_4*cos(phi_4))^2)^(1/2)) - 2*l_2*l_4*cos(phi_4))/((l_1*sin(phi_1) - l_4*sin(phi_4))^2 + (l_5 - l_1*cos(phi_1) + l_4*cos(phi_4))^2 + l_2^2 - l_3^2 + 2*l_2*(l_5 - l_1*cos(phi_1) + l_4*cos(phi_4))) - (((4*l_2^2*(l_1*sin(phi_1) - l_4*sin(phi_4))^2 - ((l_1*sin(phi_1) - l_4*sin(phi_4))^2 + (l_5 - l_1*cos(phi_1) + l_4*cos(phi_4))^2 + l_2^2 - l_3^2)^2 + 4*l_2^2*(l_5 - l_1*cos(phi_1) + l_4*cos(phi_4))^2)^(1/2) - 2*l_2*(l_1*sin(phi_1) - l_4*sin(phi_4)))*(2*l_2*l_4*sin(phi_4) + 2*l_4*cos(phi_4)*(l_1*sin(phi_1) - l_4*sin(phi_4)) + 2*l_4*sin(phi_4)*(l_5 - l_1*cos(phi_1) + l_4*cos(phi_4))))/((l_1*sin(phi_1) - l_4*sin(phi_4))^2 + (l_5 - l_1*cos(phi_1) + l_4*cos(phi_4))^2 + l_2^2 - l_3^2 + 2*l_2*(l_5 - l_1*cos(phi_1) + l_4*cos(phi_4)))^2)*(l_2*cos(2*atan(((4*l_2^2*(l_1*sin(phi_1) - l_4*sin(phi_4))^2 - ((l_1*sin(phi_1) - l_4*sin(phi_4))^2 + (l_5 - l_1*cos(phi_1) + l_4*cos(phi_4))^2 + l_2^2 - l_3^2)^2 + 4*l_2^2*(l_5 - l_1*cos(phi_1) + l_4*cos(phi_4))^2)^(1/2) - 2*l_2*(l_1*sin(phi_1) - l_4*sin(phi_4)))/((l_1*sin(phi_1) - l_4*sin(phi_4))^2 + (l_5 - l_1*cos(phi_1) + l_4*cos(phi_4))^2 + l_2^2 - l_3^2 + 2*l_2*(l_5 - l_1*cos(phi_1) + l_4*cos(phi_4))))) - l_5/2 + l_1*cos(phi_1)))/(((4*l_2^2*(l_1*sin(phi_1) - l_4*sin(phi_4))^2 - ((l_1*sin(phi_1) - l_4*sin(phi_4))^2 + (l_5 - l_1*cos(phi_1) + l_4*cos(phi_4))^2 + l_2^2 - l_3^2)^2 + 4*l_2^2*(l_5 - l_1*cos(phi_1) + l_4*cos(phi_4))^2)^(1/2) - 2*l_2*(l_1*sin(phi_1) - l_4*sin(phi_4)))^2/((l_1*sin(phi_1) - l_4*sin(phi_4))^2 + (l_5 - l_1*cos(phi_1) + l_4*cos(phi_4))^2 + l_2^2 - l_3^2 + 2*l_2*(l_5 - l_1*cos(phi_1) + l_4*cos(phi_4)))^2 + 1) - (4*l_2*cos(2*atan(((4*l_2^2*(l_1*sin(phi_1) - l_4*sin(phi_4))^2 - ((l_1*sin(phi_1) - l_4*sin(phi_4))^2 + (l_5 - l_1*cos(phi_1) + l_4*cos(phi_4))^2 + l_2^2 - l_3^2)^2 + 4*l_2^2*(l_5 - l_1*cos(phi_1) + l_4*cos(phi_4))^2)^(1/2) - 2*l_2*(l_1*sin(phi_1) - l_4*sin(phi_4)))/((l_1*sin(phi_1) - l_4*sin(phi_4))^2 + (l_5 - l_1*cos(phi_1) + l_4*cos(phi_4))^2 + l_2^2 - l_3^2 + 2*l_2*(l_5 - l_1*cos(phi_1) + l_4*cos(phi_4)))))*(l_2*sin(2*atan(((4*l_2^2*(l_1*sin(phi_1) - l_4*sin(phi_4))^2 - ((l_1*sin(phi_1) - l_4*sin(phi_4))^2 + (l_5 - l_1*cos(phi_1) + l_4*cos(phi_4))^2 + l_2^2 - l_3^2)^2 + 4*l_2^2*(l_5 - l_1*cos(phi_1) + l_4*cos(phi_4))^2)^(1/2) - 2*l_2*(l_1*sin(phi_1) - l_4*sin(phi_4)))/((l_1*sin(phi_1) - l_4*sin(phi_4))^2 + (l_5 - l_1*cos(phi_1) + l_4*cos(phi_4))^2 + l_2^2 - l_3^2 + 2*l_2*(l_5 - l_1*cos(phi_1) + l_4*cos(phi_4))))) + l_1*sin(phi_1))*(((8*l_2^2*l_4*cos(phi_4)*(l_1*sin(phi_1) - l_4*sin(phi_4)) - 2*(2*l_4*cos(phi_4)*(l_1*sin(phi_1) - l_4*sin(phi_4)) + 2*l_4*sin(phi_4)*(l_5 - l_1*cos(phi_1) + l_4*cos(phi_4)))*((l_1*sin(phi_1) - l_4*sin(phi_4))^2 + (l_5 - l_1*cos(phi_1) + l_4*cos(phi_4))^2 + l_2^2 - l_3^2) + 8*l_2^2*l_4*sin(phi_4)*(l_5 - l_1*cos(phi_1) + l_4*cos(phi_4)))/(2*(4*l_2^2*(l_1*sin(phi_1) - l_4*sin(phi_4))^2 - ((l_1*sin(phi_1) - l_4*sin(phi_4))^2 + (l_5 - l_1*cos(phi_1) + l_4*cos(phi_4))^2 + l_2^2 - l_3^2)^2 + 4*l_2^2*(l_5 - l_1*cos(phi_1) + l_4*cos(phi_4))^2)^(1/2)) - 2*l_2*l_4*cos(phi_4))/((l_1*sin(phi_1) - l_4*sin(phi_4))^2 + (l_5 - l_1*cos(phi_1) + l_4*cos(phi_4))^2 + l_2^2 - l_3^2 + 2*l_2*(l_5 - l_1*cos(phi_1) + l_4*cos(phi_4))) - (((4*l_2^2*(l_1*sin(phi_1) - l_4*sin(phi_4))^2 - ((l_1*sin(phi_1) - l_4*sin(phi_4))^2 + (l_5 - l_1*cos(phi_1) + l_4*cos(phi_4))^2 + l_2^2 - l_3^2)^2 + 4*l_2^2*(l_5 - l_1*cos(phi_1) + l_4*cos(phi_4))^2)^(1/2) - 2*l_2*(l_1*sin(phi_1) - l_4*sin(phi_4)))*(2*l_2*l_4*sin(phi_4) + 2*l_4*cos(phi_4)*(l_1*sin(phi_1) - l_4*sin(phi_4)) + 2*l_4*sin(phi_4)*(l_5 - l_1*cos(phi_1) + l_4*cos(phi_4))))/((l_1*sin(phi_1) - l_4*sin(phi_4))^2 + (l_5 - l_1*cos(phi_1) + l_4*cos(phi_4))^2 + l_2^2 - l_3^2 + 2*l_2*(l_5 - l_1*cos(phi_1) + l_4*cos(phi_4)))^2))/(((4*l_2^2*(l_1*sin(phi_1) - l_4*sin(phi_4))^2 - ((l_1*sin(phi_1) - l_4*sin(phi_4))^2 + (l_5 - l_1*cos(phi_1) + l_4*cos(phi_4))^2 + l_2^2 - l_3^2)^2 + 4*l_2^2*(l_5 - l_1*cos(phi_1) + l_4*cos(phi_4))^2)^(1/2) - 2*l_2*(l_1*sin(phi_1) - l_4*sin(phi_4)))^2/((l_1*sin(phi_1) - l_4*sin(phi_4))^2 + (l_5 - l_1*cos(phi_1) + l_4*cos(phi_4))^2 + l_2^2 - l_3^2 + 2*l_2*(l_5 - l_1*cos(phi_1) + l_4*cos(phi_4)))^2 + 1))*(l_2*cos(2*atan(((4*l_2^2*(l_1*sin(phi_1) - l_4*sin(phi_4))^2 - ((l_1*sin(phi_1) - l_4*sin(phi_4))^2 + (l_5 - l_1*cos(phi_1) + l_4*cos(phi_4))^2 + l_2^2 - l_3^2)^2 + 4*l_2^2*(l_5 - l_1*cos(phi_1) + l_4*cos(phi_4))^2)^(1/2) - 2*l_2*(l_1*sin(phi_1) - l_4*sin(phi_4)))/((l_1*sin(phi_1) - l_4*sin(phi_4))^2 + (l_5 - l_1*cos(phi_1) + l_4*cos(phi_4))^2 + l_2^2 - l_3^2 + 2*l_2*(l_5 - l_1*cos(phi_1) + l_4*cos(phi_4))))) - l_5/2 + l_1*cos(phi_1)))/(2*((l_2*sin(2*atan(((4*l_2^2*(l_1*sin(phi_1) - l_4*sin(phi_4))^2 - ((l_1*sin(phi_1) - l_4*sin(phi_4))^2 + (l_5 - l_1*cos(phi_1) + l_4*cos(phi_4))^2 + l_2^2 - l_3^2)^2 + 4*l_2^2*(l_5 - l_1*cos(phi_1) + l_4*cos(phi_4))^2)^(1/2) - 2*l_2*(l_1*sin(phi_1) - l_4*sin(phi_4)))/((l_1*sin(phi_1) - l_4*sin(phi_4))^2 + (l_5 - l_1*cos(phi_1) + l_4*cos(phi_4))^2 + l_2^2 - l_3^2 + 2*l_2*(l_5 - l_1*cos(phi_1) + l_4*cos(phi_4))))) + l_1*sin(phi_1))^2 + (l_2*cos(2*atan(((4*l_2^2*(l_1*sin(phi_1) - l_4*sin(phi_4))^2 - ((l_1*sin(phi_1) - l_4*sin(phi_4))^2 + (l_5 - l_1*cos(phi_1) + l_4*cos(phi_4))^2 + l_2^2 - l_3^2)^2 + 4*l_2^2*(l_5 - l_1*cos(phi_1) + l_4*cos(phi_4))^2)^(1/2) - 2*l_2*(l_1*sin(phi_1) - l_4*sin(phi_4)))/((l_1*sin(phi_1) - l_4*sin(phi_4))^2 + (l_5 - l_1*cos(phi_1) + l_4*cos(phi_4))^2 + l_2^2 - l_3^2 + 2*l_2*(l_5 - l_1*cos(phi_1) + l_4*cos(phi_4))))) - l_5/2 + l_1*cos(phi_1))^2)^(3/2)) - (2*l_2*sin(2*atan(((4*l_2^2*(l_1*sin(phi_1) - l_4*sin(phi_4))^2 - ((l_1*sin(phi_1) - l_4*sin(phi_4))^2 + (l_5 - l_1*cos(phi_1) + l_4*cos(phi_4))^2 + l_2^2 - l_3^2)^2 + 4*l_2^2*(l_5 - l_1*cos(phi_1) + l_4*cos(phi_4))^2)^(1/2) - 2*l_2*(l_1*sin(phi_1) - l_4*sin(phi_4)))/((l_1*sin(phi_1) - l_4*sin(phi_4))^2 + (l_5 - l_1*cos(phi_1) + l_4*cos(phi_4))^2 + l_2^2 - l_3^2 + 2*l_2*(l_5 - l_1*cos(phi_1) + l_4*cos(phi_4)))))*(((8*l_2^2*l_4*cos(phi_4)*(l_1*sin(phi_1) - l_4*sin(phi_4)) - 2*(2*l_4*cos(phi_4)*(l_1*sin(phi_1) - l_4*sin(phi_4)) + 2*l_4*sin(phi_4)*(l_5 - l_1*cos(phi_1) + l_4*cos(phi_4)))*((l_1*sin(phi_1) - l_4*sin(phi_4))^2 + (l_5 - l_1*cos(phi_1) + l_4*cos(phi_4))^2 + l_2^2 - l_3^2) + 8*l_2^2*l_4*sin(phi_4)*(l_5 - l_1*cos(phi_1) + l_4*cos(phi_4)))/(2*(4*l_2^2*(l_1*sin(phi_1) - l_4*sin(phi_4))^2 - ((l_1*sin(phi_1) - l_4*sin(phi_4))^2 + (l_5 - l_1*cos(phi_1) + l_4*cos(phi_4))^2 + l_2^2 - l_3^2)^2 + 4*l_2^2*(l_5 - l_1*cos(phi_1) + l_4*cos(phi_4))^2)^(1/2)) - 2*l_2*l_4*cos(phi_4))/((l_1*sin(phi_1) - l_4*sin(phi_4))^2 + (l_5 - l_1*cos(phi_1) + l_4*cos(phi_4))^2 + l_2^2 - l_3^2 + 2*l_2*(l_5 - l_1*cos(phi_1) + l_4*cos(phi_4))) - (((4*l_2^2*(l_1*sin(phi_1) - l_4*sin(phi_4))^2 - ((l_1*sin(phi_1) - l_4*sin(phi_4))^2 + (l_5 - l_1*cos(phi_1) + l_4*cos(phi_4))^2 + l_2^2 - l_3^2)^2 + 4*l_2^2*(l_5 - l_1*cos(phi_1) + l_4*cos(phi_4))^2)^(1/2) - 2*l_2*(l_1*sin(phi_1) - l_4*sin(phi_4)))*(2*l_2*l_4*sin(phi_4) + 2*l_4*cos(phi_4)*(l_1*sin(phi_1) - l_4*sin(phi_4)) + 2*l_4*sin(phi_4)*(l_5 - l_1*cos(phi_1) + l_4*cos(phi_4))))/((l_1*sin(phi_1) - l_4*sin(phi_4))^2 + (l_5 - l_1*cos(phi_1) + l_4*cos(phi_4))^2 + l_2^2 - l_3^2 + 2*l_2*(l_5 - l_1*cos(phi_1) + l_4*cos(phi_4)))^2))/(((l_2*sin(2*atan(((4*l_2^2*(l_1*sin(phi_1) - l_4*sin(phi_4))^2 - ((l_1*sin(phi_1) - l_4*sin(phi_4))^2 + (l_5 - l_1*cos(phi_1) + l_4*cos(phi_4))^2 + l_2^2 - l_3^2)^2 + 4*l_2^2*(l_5 - l_1*cos(phi_1) + l_4*cos(phi_4))^2)^(1/2) - 2*l_2*(l_1*sin(phi_1) - l_4*sin(phi_4)))/((l_1*sin(phi_1) - l_4*sin(phi_4))^2 + (l_5 - l_1*cos(phi_1) + l_4*cos(phi_4))^2 + l_2^2 - l_3^2 + 2*l_2*(l_5 - l_1*cos(phi_1) + l_4*cos(phi_4))))) + l_1*sin(phi_1))^2 + (l_2*cos(2*atan(((4*l_2^2*(l_1*sin(phi_1) - l_4*sin(phi_4))^2 - ((l_1*sin(phi_1) - l_4*sin(phi_4))^2 + (l_5 - l_1*cos(phi_1) + l_4*cos(phi_4))^2 + l_2^2 - l_3^2)^2 + 4*l_2^2*(l_5 - l_1*cos(phi_1) + l_4*cos(phi_4))^2)^(1/2) - 2*l_2*(l_1*sin(phi_1) - l_4*sin(phi_4)))/((l_1*sin(phi_1) - l_4*sin(phi_4))^2 + (l_5 - l_1*cos(phi_1) + l_4*cos(phi_4))^2 + l_2^2 - l_3^2 + 2*l_2*(l_5 - l_1*cos(phi_1) + l_4*cos(phi_4))))) - l_5/2 + l_1*cos(phi_1))^2)^(1/2)*(((4*l_2^2*(l_1*sin(phi_1) - l_4*sin(phi_4))^2 - ((l_1*sin(phi_1) - l_4*sin(phi_4))^2 + (l_5 - l_1*cos(phi_1) + l_4*cos(phi_4))^2 + l_2^2 - l_3^2)^2 + 4*l_2^2*(l_5 - l_1*cos(phi_1) + l_4*cos(phi_4))^2)^(1/2) - 2*l_2*(l_1*sin(phi_1) - l_4*sin(phi_4)))^2/((l_1*sin(phi_1) - l_4*sin(phi_4))^2 + (l_5 - l_1*cos(phi_1) + l_4*cos(phi_4))^2 + l_2^2 - l_3^2 + 2*l_2*(l_5 - l_1*cos(phi_1) + l_4*cos(phi_4)))^2 + 1)))/(1 - (l_2*cos(2*atan(((4*l_2^2*(l_1*sin(phi_1) - l_4*sin(phi_4))^2 - ((l_1*sin(phi_1) - l_4*sin(phi_4))^2 + (l_5 - l_1*cos(phi_1) + l_4*cos(phi_4))^2 + l_2^2 - l_3^2)^2 + 4*l_2^2*(l_5 - l_1*cos(phi_1) + l_4*cos(phi_4))^2)^(1/2) - 2*l_2*(l_1*sin(phi_1) - l_4*sin(phi_4)))/((l_1*sin(phi_1) - l_4*sin(phi_4))^2 + (l_5 - l_1*cos(phi_1) + l_4*cos(phi_4))^2 + l_2^2 - l_3^2 + 2*l_2*(l_5 - l_1*cos(phi_1) + l_4*cos(phi_4))))) - l_5/2 + l_1*cos(phi_1))^2/((l_2*sin(2*atan(((4*l_2^2*(l_1*sin(phi_1) - l_4*sin(phi_4))^2 - ((l_1*sin(phi_1) - l_4*sin(phi_4))^2 + (l_5 - l_1*cos(phi_1) + l_4*cos(phi_4))^2 + l_2^2 - l_3^2)^2 + 4*l_2^2*(l_5 - l_1*cos(phi_1) + l_4*cos(phi_4))^2)^(1/2) - 2*l_2*(l_1*sin(phi_1) - l_4*sin(phi_4)))/((l_1*sin(phi_1) - l_4*sin(phi_4))^2 + (l_5 - l_1*cos(phi_1) + l_4*cos(phi_4))^2 + l_2^2 - l_3^2 + 2*l_2*(l_5 - l_1*cos(phi_1) + l_4*cos(phi_4))))) + l_1*sin(phi_1))^2 + (l_2*cos(2*atan(((4*l_2^2*(l_1*sin(phi_1) - l_4*sin(phi_4))^2 - ((l_1*sin(phi_1) - l_4*sin(phi_4))^2 + (l_5 - l_1*cos(phi_1) + l_4*cos(phi_4))^2 + l_2^2 - l_3^2)^2 + 4*l_2^2*(l_5 - l_1*cos(phi_1) + l_4*cos(phi_4))^2)^(1/2) - 2*l_2*(l_1*sin(phi_1) - l_4*sin(phi_4)))/((l_1*sin(phi_1) - l_4*sin(phi_4))^2 + (l_5 - l_1*cos(phi_1) + l_4*cos(phi_4))^2 + l_2^2 - l_3^2 + 2*l_2*(l_5 - l_1*cos(phi_1) + l_4*cos(phi_4))))) - l_5/2 + l_1*cos(phi_1))^2))^(1/2);

T1=J11*F+J21*Tp;
T2=J12*F+J22*Tp;

== matlab function Model/支持力结算/MATLAB Function ==
  data: ax input; a_M output; ay input; az input; yaw input; pitch input; roll input
function a_M = fcn(ax,ay,az,yaw,pitch,roll)

a_M=-sin(pitch)*ax+sin(roll)*cos(pitch)*ay+cos(roll)*cos(pitch)*az;

== matlab function Model/支持力结算/MATLAB Function1 ==
  data: a_M input; a_w output; L_0 input; dL_0 input; ddL_0 input; theta input; dtheta input; ddtheta input
function a_w = fcn(a_M,L_0,dL_0,ddL_0,theta,dtheta,ddtheta)

a_w = a_M-ddL_0*cos(theta)+2*dL_0*dtheta*sin(theta)+L_0*ddtheta*sin(theta)+L_0*dtheta^2*cos(theta);

== matlab function Model/支持力结算/右 ==
  data: a_M input; a_w output; L_0 input; dL_0 input; ddL_0 input; theta input; dtheta input; ddtheta input
function a_w = fcn(a_M,L_0,dL_0,ddL_0,theta,dtheta,ddtheta)

a_w = a_M-ddL_0*cos(theta)+2*dL_0*dtheta*sin(theta)+L_0*ddtheta*sin(theta)+L_0*dtheta^2*cos(theta);
